simulink model "Quad2DSimulink"  (R2023a)
settings: Solver=VariableStepAuto  StartTime=0.0  StopTime=10.0  RelTol=1e-3
values from neighbouring files (symbols this model uses):
  params =     [Quad2D_constants.mat]
undefined symbols (not defined in the file or in its folder): b_phi, b_y, b_z, init_phi, init_y, init_z, net_force, net_torque
settings Model: Creator=m260477  LastModifiedBy=m260477

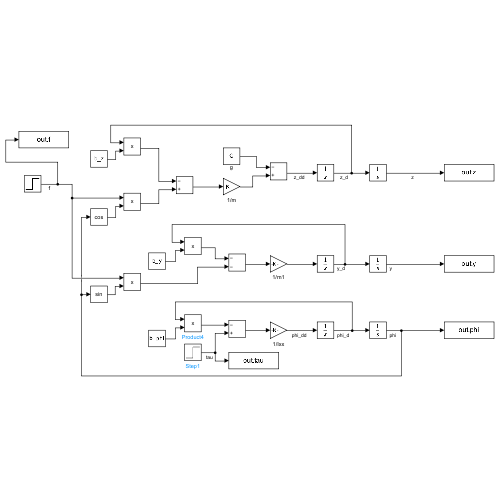
[thumbnail: Simulink's stored preview of the top-level diagram]
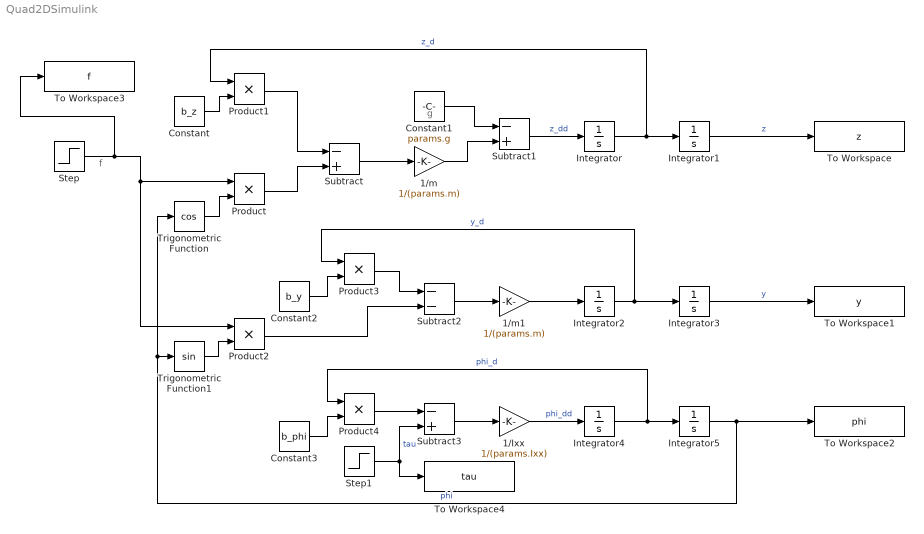
== system Quad2DSimulink ==
  note: g
  note: f
  1/Ixx : Gain  Gain=1/(params.Ixx)
  1/m : Gain  Gain=1/(params.m)
  1/m1 : Gain  Gain=1/(params.m)
  Constant : Constant  Value=b_z
  Constant1 : Constant  Value=params.g
  Constant2 : Constant  Value=b_y
  Constant3 : Constant  Value=b_phi
  Integrator : Integrator
  Integrator1 : Integrator  InitialCondition=init_z
  Integrator2 : Integrator
  Integrator3 : Integrator  InitialCondition=init_y
  Integrator4 : Integrator
  Integrator5 : Integrator  InitialCondition=init_phi
  Product{,1..4} (5 alike) : Product
  Step : Step  Time=0  After=net_force  SampleTime=0
  Step1 : Step  Time=0  After=net_torque  SampleTime=0
  Subtract : Sum  Inputs=-+
  Subtract1 : Sum  Inputs=-+
  Subtract2 : Sum  Inputs=--
  Subtract3 : Sum  Inputs=-+
  To Workspace : ToWorkspace  VariableName=z  SaveFormat=Timeseries  SampleTime=-1
  To Workspace1 : ToWorkspace  VariableName=y  SaveFormat=Timeseries  SampleTime=-1
  To Workspace2 : ToWorkspace  VariableName=phi  SaveFormat=Timeseries  SampleTime=-1
  To Workspace3 : ToWorkspace  VariableName=f  SaveFormat=Timeseries  SampleTime=-1
  To Workspace4 : ToWorkspace  VariableName=tau  SaveFormat=Timeseries  SampleTime=-1
  Trigonometric Function : Trigonometry  Operator=cos
  Trigonometric Function1 : Trigonometry
  wires:
  Integrator/1 -> Product1/1, Integrator1/1  "z_d"
  Integrator1/1 -> To Workspace/1  "z"
  Step/1 -> To Workspace3/1, Product2/1, Product/1
  Trigonometric Function/1 -> Product/2
  Product/1 -> Subtract/2
  Subtract/1 -> 1/m/1
  Subtract1/1 -> Integrator/1  "z_dd"
  1/m/1 -> Subtract1/2
  Constant1/1 -> Subtract1/1
  Constant/1 -> Product1/2
  Product1/1 -> Subtract/1
  Integrator2/1 -> Product3/1, Integrator3/1  "y_d"
  Integrator3/1 -> To Workspace1/1  "y"
  1/m1/1 -> Integrator2/1
  Trigonometric Function1/1 -> Product2/2
  Subtract2/1 -> 1/m1/1
  Constant2/1 -> Product3/2
  Product3/1 -> Subtract2/1
  Product2/1 -> Subtract2/2
  Integrator4/1 -> Product4/1, Integrator5/1  "phi_d"
  Integrator5/1 -> To Workspace2/1, Trigonometric Function/1, Trigonometric Function1/1  "phi"
  1/Ixx/1 -> Integrator4/1  "phi_dd"
  Subtract3/1 -> 1/Ixx/1
  Step1/1 -> To Workspace4/1, Subtract3/2  "tau"
  Constant3/1 -> Product4/2
  Product4/1 -> Subtract3/1
